simulink model "vab_to_uvw_test"  (R2017a)
settings: Solver=VariableStepAuto  StartTime=0.0  StopTime=10.0  RelTol=1e-3
settings Model: Creator=mudat  LastModifiedBy=mudat

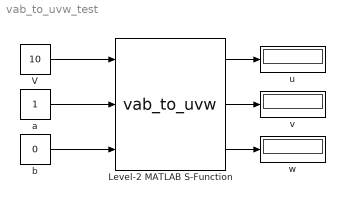
== system vab_to_uvw_test ==
  Level-2 MATLAB S-Function : M-S-Function  FunctionName=vab_to_uvw
  V : Constant  Value=10
  a : Constant
  b : Constant  Value=0
  u : Display
  v : Display
  w : Display
  wires:
  V/1 -> Level-2 MATLAB S-Function/1
  a/1 -> Level-2 MATLAB S-Function/2
  b/1 -> Level-2 MATLAB S-Function/3
  Level-2 MATLAB S-Function/1 -> u/1
  Level-2 MATLAB S-Function/2 -> v/1
  Level-2 MATLAB S-Function/3 -> w/1
